simulink model "transfer_function_2rd"  (R2019b)
settings: Solver=ode4  StartTime=0.0  StopTime=100  FixedStep=0.0001  RelTol=1e-3
libraries: simulink x1
settings Model: Creator=bitgar  LastModifiedBy=zczhu
settings DataIOCC: ReturnWorkspaceOutputs=off

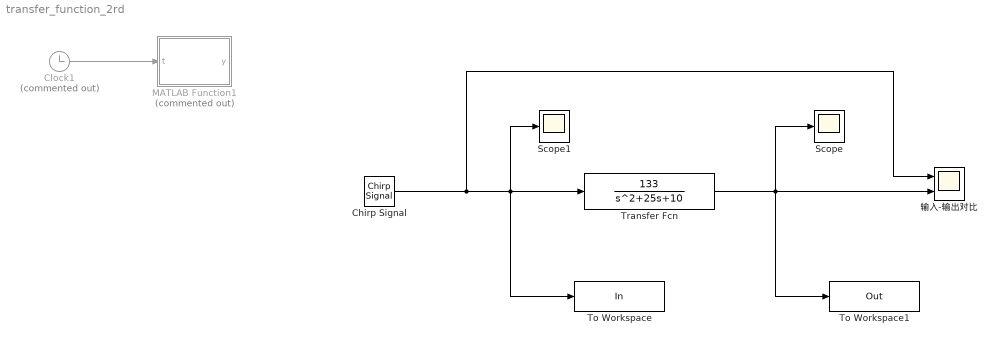
== system transfer_function_2rd ==
  Chirp Signal : simulink/Sources/Chirp Signal  f1=0.1  T=100  f2=100
  Clock1 : Clock  Commented=on
  MATLAB Function1 : MATLAB Function  Commented=on  TreatAsAtomicUnit=on  SystemSampleTime=0.0001
  Scope : Scope
  Scope1 : Scope
  To Workspace : ToWorkspace  VariableName=In  SampleTime=-1
  To Workspace1 : ToWorkspace  VariableName=Out  SampleTime=-1
  Transfer Fcn : TransferFcn  Numerator=[133]  Denominator=[1 25 10]
  输入-输出对比 : Scope  NumInputPorts=2
  wires:
  Transfer Fcn/1 -> 输入-输出对比/2, To Workspace1/1, Scope/1
  Chirp Signal/1 -> 输入-输出对比/1, Scope1/1, To Workspace/1, Transfer Fcn/1
  Clock1/1 -> MATLAB Function1/1(t)

== matlab function transfer_function_2rd/MATLAB Function1 ==
  data: t input; y output
function y = sweep_sin(t)
% sweep_sin  阶梯扫频正弦（外部时钟版）
%   t : 当前仿真时间，由 Clock 模块提供
%   y : 输出正弦，幅值=1，频率每 Tstep 升 1 Hz

% --------- 用户可改参数 ----------
Tstep = 1;          % 每 1 s 升 1 Hz（想 2 s 就改 2）
f0    = 1;          % 起始频率 0 Hz
% ----------------------------------

persistent t0 f phase0
if isempty(t0)
    t0 = 0;         % 本段起始时间
    f  = f0;        % 当前频率
    phase0 = 0;     % 本段初始相位
end

% 该换段了？
if t - t0 >= Tstep
    phase0 = phase0 + 2*pi*f*(Tstep);   % 累加相位
    t0     = t;                         % 重置段起点
    f      = f + 1;                     % 升 1 Hz
end

% 本段内连续正弦
y = sin(phase0 + 2*pi*f*(t - t0));
